simulink model "trayectoria_prueba"  (R2021a)
settings: Solver=FixedStepAuto  StartTime=0.0  StopTime=80  FixedStep=1e-3  RelTol=1e-3
libraries: simulink_extras x1
settings Model: Creator=agustin  LastModifiedBy=agustin

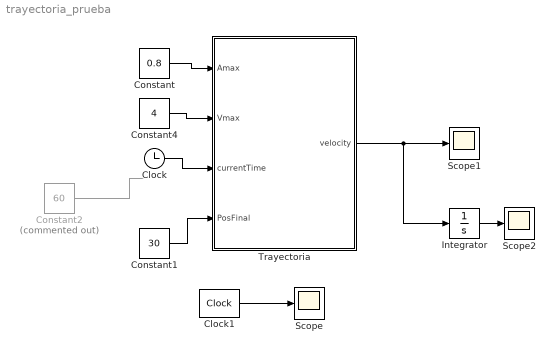
== system trayectoria_prueba ==
  Clock : Clock
  Clock1 : simulink_extras/Flip Flops/Clock  period=2e-3
  Constant : Constant  Value=0.8
  Constant1 : Constant  Value=30
  Constant2 : Constant  Commented=on  Value=60
  Constant4 : Constant  Value=4
  Integrator : Integrator
  Scope : Scope
  Scope1 : Scope
  Scope2 : Scope
  Trayectoria : Stateflow chart  TreatAsAtomicUnit=on
  wires:
  Clock1/1 -> Scope/1
  Trayectoria/1(velocity) -> Integrator/1, Scope1/1
  Constant4/1 -> Trayectoria/2(Vmax)
  Clock/1 -> Trayectoria/3(currentTime)
  Constant/1 -> Trayectoria/1(Amax)
  Constant1/1 -> Trayectoria/4(PosFinal)
  Integrator/1 -> Scope2/1
  Constant2/1 -> ?

== stateflow chart trayectoria_prueba/Trayectoria ==
  state trayectoria [commented out]
    entry:
    % Número de muestras
    %num_samples = floor(tTotal / sampleTime);
    %velocityProfile = zeros(1,num_samples);
    [velocityProfile] = generateVelocityProfile(vMax, aMax, tTotal, sampleTime);
    during:
    %En el estado donde recorres el vector de trayectoria
    index = 1; % Inicializa el índice
    while index < length(velocityProfile)
    current_position = velocityProfile(index); % Accede al elemento actual
    %Hacer algo con current_position, como controlar la velocidad
    index = index + 1; % Incrementa el índice
    end
  state INI [commented out]
    entry:
    initialTime = 0;
  state trayectoria1
    entry:
    initialTime = 10; %currentTime;
    % perfil de velocidad teniendo en cuenta el tiempo, no el espacio a alcanzar
    % totalTime: tiempo necesario para llegar al x final
    totalTime = calcularTiempoTrapezoidal(PosFinal, Vmax, Amax);
    velocity = generateVelocityProfile(Vmax, Amax, currentTime, totalTime, initialTime);
    during:
    velocity = generateVelocityProfile(Vmax, Amax, currentTime, totalTime, initialTime);
  state reachedSetPoint [commented out]
    entry:
    velocity =0;
    during:
    velocity =0;
  (default) -> trayectoria [commented out]
  INI -> trayectoria1 [commented out] : [estado == 2]
  (default) -> trayectoria1
  trayectoria1 -> reachedSetPoint [commented out] : [estado == 5]
  data: v_max function_input; a_max function_input; t_total function_input; sample_time function_input; velocity_profile function_output; v_max function_input; a_max function_input; current_time function_input; total_time function_input; next_velocity function_output; initial_time function_input; posicion_final function_input; velocidad_maxima function_input; aceleracion_maxima function_input; tiempo function_output; index local; velocityProfile local double; num_samples local; Amax input; Vmax input; currentTime input; velocity output; initialTime local; PosFinal input; totalTime local
  function velocity_profile = generateVelocityProfile(v_max, a_max, t_total, sample_time):
    | function velocity_profile = generateVelocityProfile(v_max, a_max, t_total, sample_time)
    |     % Parámetros de tiempo
    |     t_acceleration = v_max / a_max;  % Tiempo de aceleración para alcanzar v_max
    |     t_constant = (t_total - 2 * t_acceleration);  % Tiempo en velocidad constante
    |     t_deceleration = t_acceleration;  % Tiempo de desaceleración para llegar a 0
    | 
    |     % Número de muestras
    |     num_samples = floor(t_total / sample_time);
    | 
    |     % Vector de tiempos
    |     time = (0:num_samples) * sample_time;
    | 
    |     % Vector de velocidades
    |     velocity_profile = zeros(size(time));
    | 
    |     % Generar el perfil de velocidad
    |     for i = 1:length(time)
    |         if time(i) < t_acceleration
    |             velocity_profile(i) = a_max * time(i);
    |         elseif time(i) < (t_acceleration + t_constant)
    |             velocity_profile(i) = v_max;
    |         else
    |             velocity_profile(i) = v_max - a_max * (time(i) - t_acceleration - t_constant);
    |         end
    |     end
    | end
  function next_velocity = generateVelocityProfile(v_max, a_max, current_time, total_time, initial_time):
    | function next_velocity = generateVelocityProfile(v_max, a_max, current_time, total_time, initial_time)
    |     % Parámetros de tiempo
    |     t_acceleration = v_max / a_max;  % Tiempo de aceleración para alcanzar v_max
    |     t_constant = (total_time - 2 * t_acceleration);  % Tiempo en velocidad constante
    |     
    |     % Ajuste el tiempo actual para tener en cuenta el tiempo inicial
    |     current_time_adjusted = current_time - initial_time;
    |     if current_time_adjusted <= 0
    |         next_velocity = 0;
    |     elseif current_time_adjusted <= t_acceleration
    |         next_velocity = a_max * current_time_adjusted;
    |     elseif current_time_adjusted > t_acceleration && current_time_adjusted < (total_time - t_acceleration)
    |         next_velocity = v_max;
    |     else
    |         time_in_deceleration = total_time - current_time_adjusted;
    |         if time_in_deceleration < 0
    |             next_velocity = 0;
    |         else
    |             next_velocity = v_max - a_max * (current_time_adjusted - t_acceleration - t_constant);
    |         end
    |     end
    | end
    | 
    | % function next_velocity = generateVelocityProfile(v_max, a_max, current_time, total_time)
    | %     % Parámetros de tiempo
    | %     t_acceleration = v_max / a_max;  % Tiempo de aceleración para alcanzar v_max
    | %     t_constant = (total_time - 2 * t_acceleration);  % Tiempo en velocidad constante
    | %     if current_time <= t_acceleration
    | %         next_velocity = a_max * current_time;
    | %     elseif current_time > t_acceleration && current_time < (total_time - t_acceleration)
    | %         next_velocity = v_max;
    | %     else
    | %         time_in_deceleration = total_time - current_time;
    | %         if time_in_deceleration < 0
    | %             next_velocity = 0;
    | %         else
    | %             next_velocity = v_max - a_max * (current_time - t_acceleration - t_constant);
    | %             %tiempo de desaceleracion: tiempo total - tiempo total acel - tiempo cte 
    | %         end
    | %     end
    | % end
  function tiempo = calcularTiempoTrapezoidal(posicion_final, velocidad_maxima, aceleracion_maxima):
    | function tiempo = calcularTiempoTrapezoidal(posicion_final, velocidad_maxima, aceleracion_maxima)
    |     % Calcula el tiempo necesario para una trayectoria trapezoidal
    |     
    |     % Verifica si la velocidad máxima es alcanzable con la aceleración máxima
    |     tiempo_aceleracion = velocidad_maxima / aceleracion_maxima;
    |     distancia_aceleracion = 0.5 * velocidad_maxima * tiempo_aceleracion;
    |     
    |     % Calcula el tiempo necesario para desacelerar desde la velocidad máxima
    |     tiempo_desaceleracion = velocidad_maxima / aceleracion_maxima;
    |     
    |     % Calcula la distancia total a recorrer
    |     distancia_total = abs(posicion_final);
    |     
    |     if distancia_total <= 2 * distancia_aceleracion
    |         % No se alcanza la velocidad máxima, la aceleración es limitante
    |         tiempo = sqrt(distancia_total / aceleracion_maxima);
    |     else
    |         % Se alcanza la velocidad máxima
    |         tiempo = tiempo_aceleracion + (distancia_total - 2 * distancia_aceleracion) / velocidad_maxima + tiempo_desaceleracion;
    |     end
    | end
